simulink model "BiCopter"  (R2016a)
settings: Solver=VariableStepAuto  StartTime=0.0  StopTime=10.0  RelTol=1e-3
values from neighbouring files (symbols this model uses):
  g = 9.81    [BiCopter_HeightOnly.m]    (also in BiCopter_script.m)
  I = m/12 * (L^2 + H^2)    (= 0.108333333333)    [BiCopter_HeightOnly.m]    (also in BiCopter_script.m = 0.0108333333333)
  L = 0.5    [BiCopter_HeightOnly.m]    (also in BiCopter_script.m)
  m = 5    [BiCopter_HeightOnly.m]    (also in BiCopter_script.m = 0.5)
  r = 2    [BiCopter_HeightOnly.m]    (also in BiCopter_script.m = [0; 10])
settings Model: Creator=Austin  LastModifiedBy=Austin
settings DataIOCC: Refine=5

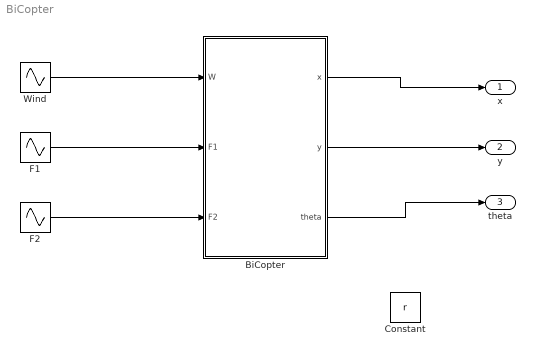
== system BiCopter ==
  BiCopter : Subsystem
  Constant : Constant  Value=r
  F1 : Sin  Amplitude=0.5  Bias=0.6*m*g  Frequency=10  Phase=pi/2  SampleTime=0
  F2 : Sin  Amplitude=0.5  Bias=0.6*m*g  Frequency=10  SampleTime=0
  Wind : Sin  Amplitude=0  Frequency=2  Phase=pi/2  SampleTime=0
  x : Outport
  y : Outport  Port=2
  theta : Outport  Port=3
  wires:
  BiCopter/1(x) -> x/1
  BiCopter/2(y) -> y/1
  BiCopter/3(theta) -> theta/1
  Wind/1 -> BiCopter/1(W)
  F1/1 -> BiCopter/2(F1)
  F2/1 -> BiCopter/3(F2)

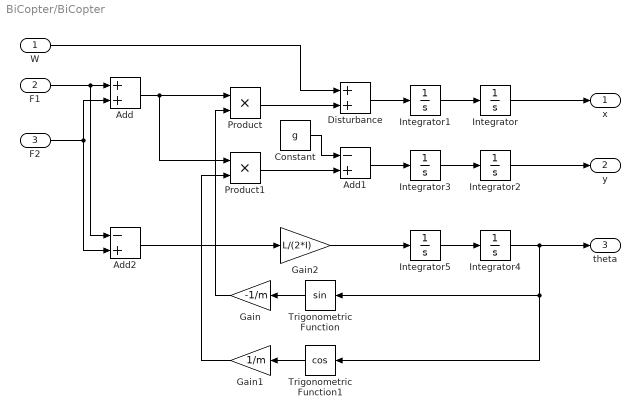
== system BiCopter/BiCopter ==
  W : Inport
  F1 : Inport  Port=2
  F2 : Inport  Port=3
  Add : Sum
  Add1 : Sum  Inputs=-+
  Add2 : Sum  Inputs=-+
  Constant : Constant  Value=g
  Disturbance : Sum
  Gain : Gain  Gain=-1/m
  Gain1 : Gain  Gain=1/m
  Gain2 : Gain  Gain=L/(2*I)
  Integrator{,1..5} (6 alike) : Integrator
  Product : Product
  Product1 : Product
  Trigonometric Function : Trigonometry
  Trigonometric Function1 : Trigonometry  Operator=cos
  x : Outport
  y : Outport  Port=2
  theta : Outport  Port=3
  wires:
  Integrator1/1 -> Integrator/1
  Integrator3/1 -> Integrator2/1
  Integrator2/1 -> y/1
  Add/1 -> Product1/1, Product/1
  Add2/1 -> Gain2/1
  Product1/1 -> Add1/2
  Add1/1 -> Integrator3/1
  Trigonometric Function/1 -> Gain/1
  Trigonometric Function1/1 -> Gain1/1
  Gain/1 -> Product/2
  Constant/1 -> Add1/1
  Gain2/1 -> Integrator5/1
  Gain1/1 -> Product1/2
  F1/1 -> Add2/1, Add/1
  Integrator/1 -> x/1
  Integrator4/1 -> theta/1, Trigonometric Function1/1, Trigonometric Function/1
  Integrator5/1 -> Integrator4/1
  F2/1 -> Add/2, Add2/2
  Product/1 -> Disturbance/2
  W/1 -> Disturbance/1
  Disturbance/1 -> Integrator1/1
